simulink model "j4s"  (R2023b)
settings: Solver=FixedStepAuto  StartTime=0.0  StopTime=10  FixedStep=0.001  RelTol=1e-3
values from neighbouring files (symbols this model uses):
  dy0 = -1.04935751    [j4.m]
settings Model: Creator=asus  LastModifiedBy=asus

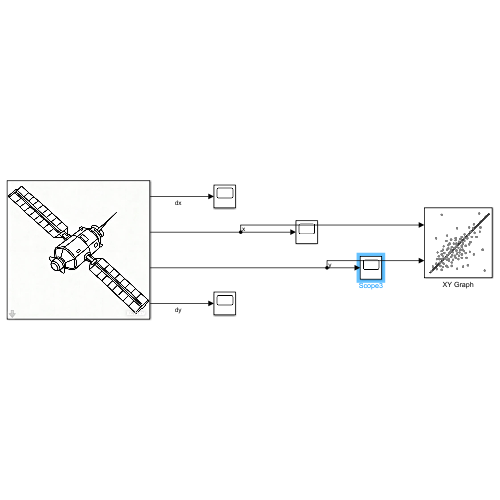
[thumbnail: Simulink's stored preview of the top-level diagram]
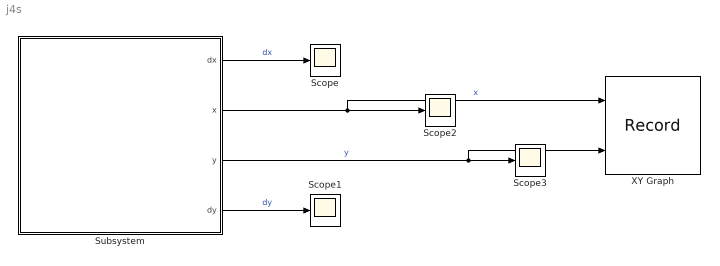
== system j4s ==
  Scope{,1..3} (4 alike) : Scope
  Subsystem : Subsystem  mask{u=1 / 82.45, x0=1.2, dx0=0, y0=0, Parameter5=-1.04935751}
      mask prompts: x0 "x(0)"; dx0 "\dot{x}(0)"; y0 "y(0)"; Parameter5 "\dot{y}(0)"
      mask DialogControl ParameterGroupVar Prompt: 参数
      mask Display: image('9f70da94fb302195e8cc36828a960293.jpg');
  XY Graph : Record  FileSettingsInternal="{\"entries\":[{\"content\":{\"excelSettings\":{\"content\":{},\"type\":\"Streamout.ExcelSettings\"}},\"type\":\"Streamout.FileSettingStorage\",\"uuid\":\"\"}],\"packageUris\":[\"http:\\/\\/schema.mathworks.com\\/mf0\\/streamout_blocks\\/R2020a\"],\"version\":\"1.0\"}"  Layout=[1 1]  SignalsInternal="{\"entries\":[{\"content\":{\"signals\":[{\"content\":{\"blockPath\":[],\"dimensions\":[1],\"domain\":\"\",\"lineColor\":\"#a2142f\",\"plots\":[1],\"port\":1,\"sid\":[\"\"],\"signalID\":270,\"signalName\":\"x\"},\"type\":\"RecordBlkView.Signal\",\"uuid\":\"\"},{\"content\":{\"blockPath\":[],\"dimensions\":[1],\"domain\":\"\",\"lineColor\":\"#139fff\",\"plots\":[1],\"port\":2,\"sid\":[\"\"],\"signalID\":274,\"signalName\":\"y\"},\"type\":\"RecordBlkView.Signal\",\"uuid\":\"\"}]},\"type\":\"RecordBlkView.InputSignals\",\"uuid\":\"\"}],\"packageUris\":[\"http:\\/\\/schema.mathworks.com\\/mf0\\/streamout_blocks\\/R2020a\"],\"version\":\"1.0\"}"  VisualizationBindings="{\"xyplotplugin\":{\"info\":[{\"series\":[{\"bindingParametersList\":[{\"parameter\":\"X-Axis\",\"signalID\":270,\"signalName\":\"x\"},{\"parameter\":\"Y-Axis\",\"signalID\":274,\"signalName\":\"y\"}],\"seriesID\":10454}],\"subplotID\":1}]}}"  CompatibilityTag=XY
  wires:
  Subsystem/1(dx) -> Scope/1  "dx"
  Subsystem/2(x) -> Scope2/1, XY Graph/1  "x"
  Subsystem/3(y) -> Scope3/1, XY Graph/2  "y"
  Subsystem/4(dy) -> Scope1/1  "dy"

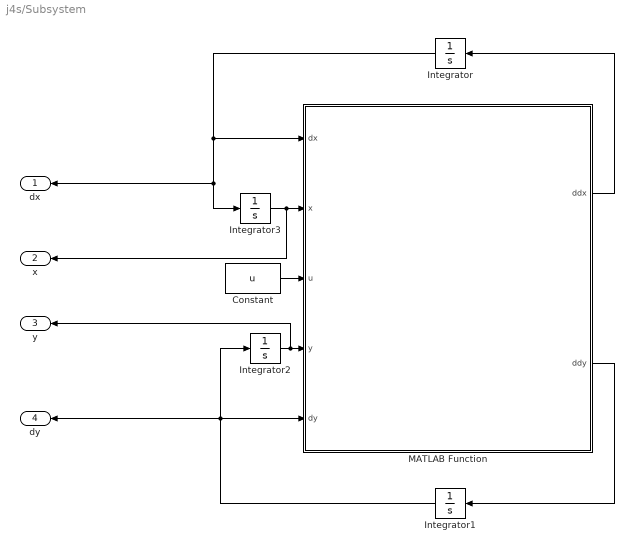
== system j4s/Subsystem ==
  Constant : Constant  Value=u
  Integrator : Integrator  InitialCondition=dx0
  Integrator1 : Integrator  InitialCondition=dy0
  Integrator2 : Integrator  InitialCondition=y0
  Integrator3 : Integrator  InitialCondition=x0
  MATLAB Function : MATLAB Function  TreatAsAtomicUnit=on
  dx : Outport
  x : Outport  Port=2
  y : Outport  Port=3
  dy : Outport  Port=4
  wires:
  Integrator/1 -> MATLAB Function/1(dx), dx/1, Integrator3/1
  Constant/1 -> MATLAB Function/3(u)
  Integrator3/1 -> x/1, MATLAB Function/2(x)
  MATLAB Function/1(ddx) -> Integrator/1
  Integrator1/1 -> dy/1, Integrator2/1, MATLAB Function/5(dy)
  Integrator2/1 -> y/1, MATLAB Function/4(y)
  MATLAB Function/2(ddy) -> Integrator1/1

== matlab function j4s/Subsystem/MATLAB Function ==
  data: dx input; x input; u input; y input; dy input; ddx output; ddy output
function [ddx,ddy] = fcn(dx,x,u,y,dy)
ux = 1 - u;
r1 = sqrt( (x + u)^2 + y^2 );
r2 = sqrt( (x - ux)^2 + y^2 );

ddx = 2*dy + x - ux*(x + u) / (r1^3) - u*(x - ux) / (r2^3);
ddy = -2*dx + y - ux*y / (r1^3) - u*y / (r2^3);
